simulink subsystem "powermanagement"  (R2022b)
settings: Solver=VariableStepAuto  StartTime=0.0  StopTime=10.0  RelTol=1e-3
libraries: simulink x1, autolibutils x1
settings Model: Creator=serga  LastModifiedBy=serga

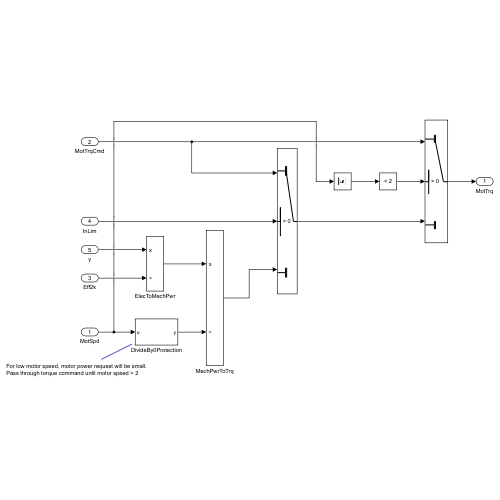
[thumbnail: Simulink's stored preview of the top-level diagram]
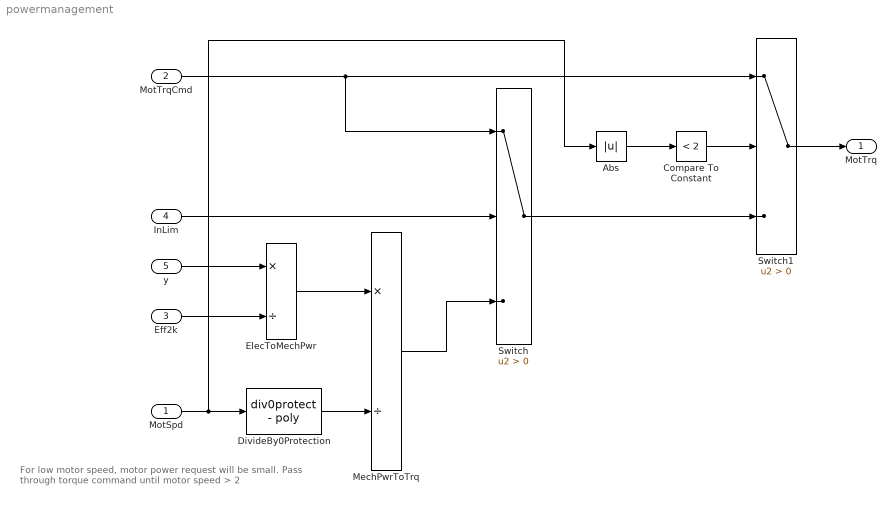
== system powermanagement ==
  note: For low motor speed, motor power request will be small. Pass through torque command until motor speed > 2
  MotSpd : Inport
  MotTrqCmd : Inport  Port=2
  Eff2k : Inport  Port=3
  InLim : Inport  Port=4
  y : Inport  Port=5
  Abs : Abs  SaturateOnIntegerOverflow=off
  Compare To Constant : simulink/Logic and Bit Operations/Compare To Constant  relop=<  const=2  OutDataTypeStr=boolean
  DivideBy0Protection : autolibutils/div0protect - poly  thresh=2  ZeroCross1=off  aMode=aMode
  ElecToMechPwr : Product  Inputs=*/
  MechPwrToTrq : Product  Inputs=*/
  Switch : Switch  Criteria=u2 > Threshold  SaturateOnIntegerOverflow=off  InputSameDT=off
  Switch1 : Switch  Criteria=u2 > Threshold  SaturateOnIntegerOverflow=off  InputSameDT=off
  MotTrq : Outport
  wires:
  y/1 -> ElecToMechPwr/1
  Eff2k/1 -> ElecToMechPwr/2
  ElecToMechPwr/1 -> MechPwrToTrq/1
  MotSpd/1 -> Abs/1, DivideBy0Protection/1
  DivideBy0Protection/1 -> MechPwrToTrq/2
  InLim/1 -> Switch/2
  MechPwrToTrq/1 -> Switch/3
  MotTrqCmd/1 -> Switch1/1, Switch/1
  Switch/1 -> Switch1/3
  Abs/1 -> Compare To Constant/1
  Compare To Constant/1 -> Switch1/2
  Switch1/1 -> MotTrq/1
